simulink model "pfb_fir"  (Simulink 7.0)
settings: Solver=FixedStepDiscrete  SolverMode=SingleTasking  StartTime=0.0  StopTime=10.0  RelTol=1e-3
undefined symbols (not defined in the file): pfb_coefs
libraries: xbsIndex_r4 x385
(part 19 of 27)

== system pfb_fir/fir_2/fir_tap_3/fir_coef ==
  data_in : Inport  OutDataType=sfix(16)  OutScaling=2^0
  sum_in : Inport  Port=2  OutDataType=sfix(16)  OutScaling=2^0
  sync_in : Inport  Port=3  OutDataType=sfix(16)  OutScaling=2^0
  c_gen : Subsystem  mask(Coefficient Generator){coefs=[0.999999547662946;0.999995928971626;0.999988691616268;0.999977835651433;0.999963361158965;0.999945268247983;0.999923557054889;0.99989822774336;0.999869280504348;0.999836715556079;0.999800533144051;0.99976073354103;0.999717317047049;0.999670283989403;0.999619634722648;0.999565369628596;0.999507489116311;0.999445993622108;0.999380883609544;0.999312159569415;0.999239822019754;0.999163871505822;0.999084308600105;0.999001133902306;0.998914348039344;0.998823951665339;0.998729945461616;0.99863233013669;0.998531106426262;0.998426275093213;0.998317836927595;0.998205792746621;0.998090143394661;0.997970889743233;0.99784803269099;0.997721573163716;0.997591512114315;0.997457850522799;0.997320589396285;0.997179729768976;0.997035272702159;0.99688721928419;0.996735570630482;0.996580327883498;0.996421492212737;0.996259064814724;0.996093046912996;0.99592343975809;0.995750244627533;0.995573462825828;0.99539309568444;0.995209144561783;0.995021610843209;0.994830495940991;0.99463580129431;0.994437528369243;0.994235678658745;0.994030253682635;0.993821254987582;0.993608684147091;0.993392542761483;0.993172832457882;0.992949554890201;0.99272271173912;0.992492304712073;0.992258335543232;0.992020805993488;0.991779717850431;0.991535072928337;0.991286873068149;0.991035120137455;0.990779816030475;0.990520962668036;0.990258561997559;0.989992615993036;0.989723126655011;0.989450096010561;0.989173526113274;0.988893419043231;0.988609776906985;0.988322601837537;0.98803189599432;0.987737661563173;0.987439900756322;0.987138615812356;0.986833808996206;0.986525482599124;0.986213638938657;0.985898280358627;0.985579409229105;0.98525702794639;0.984931138932984;0.984601744637569;0.984268847534979;0.98393245012618;0.983592554938246;0.983249164524326;0.98290228146363;0.982551908361392;0.982198047848854;0.981840702583234;0.9814798752477;0.981115568551347;0.980747785229165;0.980376528042017;0.98000179977661;0.979623603245462;0.979241941286885;0.978856816764947;0.978468232569446;0.978076191615887;0.977680696845445;0.977281751224942;0.976879357746813;0.97647351942908;0.976064239315321;0.975651520474639;0.975235366001631;0.97481577901636;0.974392762664321;0.973966320116415;0.973536454568909;0.973103169243412;0.972666467386842;0.972226352271389;0.971782827194488;0.971335895478783;0.970885560472097;0.970431825547395;0.969974694102756;0.969514169561332;0.969050255371323;0.968582955005935;0.96811227196335;0.967638209766689;0.967160771963981;0.966679962128122;0.966195783856846;0.965708240772684;0.965217336522932;0.964723074779614;0.964225459239442;0.963724493623787;0.963220181678634;0.962712527174551;0.962201533906649;0.961687205694544;0.961169546382321;0.960648559838497;0.960124249955978;0.959596620652025;0.959065675868214;0.958531419570396;0.95799385574866;0.957452988417292;0.956908821614734;0.956361359403548;0.955810605870372;0.955256565125884;0.954699241304754;0.954138638565613;0.953574761091004;0.953007613087343;0.952437198784881;0.951863522437655;0.951286588323455;0.950706400743774;0.950122964023769;0.949536282512219;0.948946360581481;0.948353202627446;0.947756813069498;0.947157196350468;0.946554356936591;0.945948299317464;0.945339028005997;0.944726547538374;0.944110862474005;0.943491977395482;0.942869896908532;0.942244625641977;0.941616168247679;0.940984529400506;0.940349713798277;0.939711726161716;0.939070571234412;0.938426253782768;0.937778778595951;0.937128150485851;0.936474374287031;0.935817454856679;0.935157397074559;0.934494205842967;0.933827886086677;0.933158442752899;0.932485880811225;0.931810205253583;0.931131421094187;0.930449533369489;0.929764547138127;0.929076467480875;0.928385299500598;0.927691048322198;0.92699371909256;0.926293316980511;0.925589847176761;0.924883314893854;0.924173725366119;0.923461083849616;0.922745395622088;0.922026665982904;0.92130490025301;0.920580103774877;0.919852281912448;0.919121440051086;0.918387583597519;0.91765071797979;0.9169108486472;0.916167981070258;0.915422120740627;0.914673273171068;0.913921443895387;0.913166638468382 ...(+14460 chars)], n_bits=9, bin_pt=8, log2_cpc=0, use_bram=on}
      mask prompts: coefs "Coefficients"; n_bits "Number of Bits"; bin_pt "Binary Point"; log2_cpc "Log2 Cycles per Coefficient"; use_bram "Use BRAM"
      mask help: A coefficient generator.
      settings: AttributesFormatString=|
      | 1024 coefs in bram
      | 9_8 out/1
      mask Help:
      | <pre>
      | Description::
      | 
      | A coefficient generator.
      | 
      | Mask Parameters::
      | 
      | Coefficiants (coefs): The coefficients to output.  These should be specified as doubles.
      | They will be rounded/saturated according to the specified number of bits (n_bits)
      | and binary point (bin_pt).
      | 
      | Number of Coefficient Bits (n_bits): The number of bits used for the fixed point binary
      | representation of the coefficients.
      | 
      | Coefficient Binary Point (bin_pt): The binary point of the fixed point binary representation
      | of the coefficients.
      | 
      | Log2 Cycles per Coefficient (log2_cpc): The log2 value of the number of cycles per coefficient.
      | Must be a non-negative integer (i.e. cycles per coefficient must be a power of 2).
      | 
      | Use BRAM (use_bram): Check this checkbox to store coefficients in BRAM.
      | If unchecked, the coefficients will be sored in distributed memory (i.e. slices).
      | </pre>
  data_delay : xbsIndex_r4/Delay  en=off  latency=1  dbl_ovrd=off  reg_retiming=off  block_type=delay
      settings: xl_area=[0, 0, 0, 0, 0, 0, 0]
  sum_delay : xbsIndex_r4/Delay  en=off  latency=1  dbl_ovrd=off  reg_retiming=off  block_type=delay
      settings: xl_area=[0, 0, 0, 0, 0, 0, 0]
  sync_delay : xbsIndex_r4/Delay  en=off  latency=1  dbl_ovrd=off  reg_retiming=off  block_type=delay
      settings: xl_area=[0, 0, 0, 0, 0, 0, 0]
  data_out : Outport  OutDataType=sfix(16)  OutScaling=2^0
  sum_out : Outport  Port=2  OutDataType=sfix(16)  OutScaling=2^0
  coef : Outport  Port=3  OutDataType=sfix(16)  OutScaling=2^0
  sync_out : Outport  Port=4  OutDataType=sfix(16)  OutScaling=2^0
  wires:
  c_gen/1(coef_out) -> coef/1
  sum_delay/1 -> sum_out/1
  sum_in/1 -> sum_delay/1
  sync_in/1 -> c_gen/1(sync_in), sync_delay/1
  sync_delay/1 -> sync_out/1
  data_delay/1 -> data_out/1
  data_in/1 -> data_delay/1

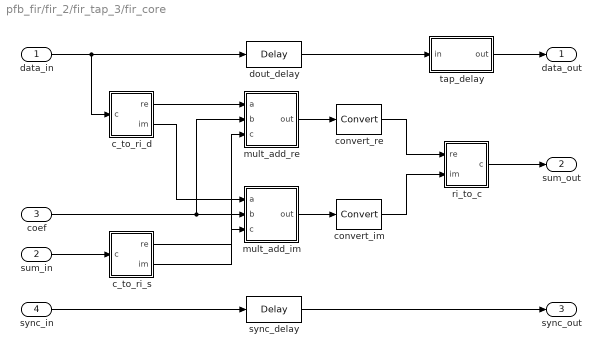
== system pfb_fir/fir_2/fir_tap_3/fir_core ==
  data_in : Inport  OutDataType=sfix(16)  OutScaling=2^0
  sum_in : Inport  Port=2  OutDataType=sfix(16)  OutScaling=2^0
  coef : Inport  Port=3  OutDataType=sfix(16)  OutScaling=2^0
  sync_in : Inport  Port=4  OutDataType=sfix(16)  OutScaling=2^0
  c_to_ri_d : Subsystem  mask(Complex to Real-Imag){n_bits=8, bin_pt=7}
      mask prompts: n_bits "Bit Width"; bin_pt "Binary Point"
      mask help: Outputs real and imaginary components of a complex input.
      settings: AttributesFormatString=8_7 r/i
      mask Help:
      | <pre>
      | Description::
      | 
      | Outputs real and imaginary components of a complex input.
      | Useful for simplifying interconnects.
      | See also: Real-Imag to Complex (ri_to_c)
      | 
      | Mask Parameters::
      | 
      | Bit Width (n_bits): Specifies the width of the real/imaginary components.
      | Assumed equal for both components.
      | 
      | Binary Point (bin_pt): Specifies the binary point location in the real/imaginary components.
      | Assumed equal for both components.
      | </pre>
  c_to_ri_s : Subsystem  mask(Complex to Real-Imag){n_bits=17, bin_pt=15}
      mask prompts: n_bits "Bit Width"; bin_pt "Binary Point"
      mask help: Outputs real and imaginary components of a complex input.
      settings: AttributesFormatString=17_15 r/i
      mask Help:
      | <pre>
      | Description::
      | 
      | Outputs real and imaginary components of a complex input.
      | Useful for simplifying interconnects.
      | See also: Real-Imag to Complex (ri_to_c)
      | 
      | Mask Parameters::
      | 
      | Bit Width (n_bits): Specifies the width of the real/imaginary components.
      | Assumed equal for both components.
      | 
      | Binary Point (bin_pt): Specifies the binary point location in the real/imaginary components.
      | Assumed equal for both components.
      | </pre>
  convert_im : xbsIndex_r4/Convert  arith_type="Signed  (2's comp)"  n_bits=17  bin_pt=15  quantization=Truncate  overflow=Wrap  latency=0  dbl_ovrd=off  pipeline=on  block_type=convert
      settings: xl_area=[0, 0, 0, 0, 0, 0, 0]  block_version=10.1.3
  convert_re : xbsIndex_r4/Convert  arith_type="Signed  (2's comp)"  n_bits=17  bin_pt=15  quantization=Truncate  overflow=Wrap  latency=0  dbl_ovrd=off  pipeline=on  block_type=convert
      settings: xl_area=[0, 0, 0, 0, 0, 0, 0]  block_version=10.1.3
  dout_delay : xbsIndex_r4/Delay  en=off  latency=4  dbl_ovrd=off  reg_retiming=off  block_type=delay
      settings: xl_area=[0, 0, 0, 0, 0, 0, 0]
  mult_add_im : Subsystem  mask(Multiply Add Block){mult_latency=3, add_latency=1, add_bypass=off}
      mask prompts: mult_latency "Multiplier Latency"; add_latency "Adder Latency"; add_bypass "Bypass Adder"
      mask help: A full precision multiply-add block. Produces a*b+c at its ab_c output. The add operation can be optionally bypassed.
      settings: AttributesFormatString=|
      | out = a*b+c
      | latency = 4
      mask Help:
      | <pre>
      | Description::
      | 
      | This full precision multiply-add block produces a*b+c at its ab_c output.
      | The add operation can be optionally bypassed.
      | 
      | Latency is one multiplier latency plus one adder latency (if not bypassing adder).
      | 
      | Mask Parameters::
      | 
      | Multiplier Latency (mult_latency): Latency to use for the underlying real multipliers.
      | 
      | Adder Latency (add_latency): Latency to use for the underlying real adders.
      | 
      | Bypass Adder (add_bypass): Check this checkbox to bypass the adder.
      | </pre>
  mult_add_re : Subsystem  mask(Multiply Add Block){mult_latency=3, add_latency=1, add_bypass=off}
      mask prompts: mult_latency "Multiplier Latency"; add_latency "Adder Latency"; add_bypass "Bypass Adder"
      mask help: A full precision multiply-add block. Produces a*b+c at its ab_c output. The add operation can be optionally bypassed.
      settings: AttributesFormatString=|
      | out = a*b+c
      | latency = 4
      mask Help:
      | <pre>
      | Description::
      | 
      | This full precision multiply-add block produces a*b+c at its ab_c output.
      | The add operation can be optionally bypassed.
      | 
      | Latency is one multiplier latency plus one adder latency (if not bypassing adder).
      | 
      | Mask Parameters::
      | 
      | Multiplier Latency (mult_latency): Latency to use for the underlying real multipliers.
      | 
      | Adder Latency (add_latency): Latency to use for the underlying real adders.
      | 
      | Bypass Adder (add_bypass): Check this checkbox to bypass the adder.
      | </pre>
  ri_to_c : Subsystem  mask(Real-Imag to Complex){}
      mask help: Concatenates real and imaginary inputs into a complex output.
      mask init:
      | ri_to_c_init(gcb);
      mask Help:
      | <pre>
      | Description::
      | 
      | Concatenates a real and imaginary input into a complex output.
      | Useful for simplifying interconnects.
      | See also: Complex to Real-Imag (c_to_ri)
      | 
      | Mask Parameters::
      | 
      | (N/A)
      | </pre>
  sync_delay : xbsIndex_r4/Delay  en=off  latency=4  dbl_ovrd=off  reg_retiming=off  block_type=delay
      settings: xl_area=[0, 0, 0, 0, 0, 0, 0]
  tap_delay : Subsystem  mask(BRAM Delay){delay_depth=1024, buffer_latency=}
      mask prompts: delay_depth "Delay Depth"; buffer_latency "Buffer Latency"
      mask help: A delay block that uses BRAM for its storage.
      settings: AttributesFormatString=bram depth = 1024
      mask Help:
      | <pre>
      | Description::
      | 
      | A delay block that uses BRAM for its storage.
      | 
      | Mask Parameters::
      | 
      | Delay Depth (delay_depth): The length of the delay.
      | 
      | Buffer Latency (buffer_latency): The latency of the underlying storage.
      | 
      | Buffer Latency defaults to 1 and cannot be changed via the block's dialog box.
      | Future versions may enable the setting of that parameter from the dialog.
      | </pre>
  data_out : Outport  OutDataType=sfix(16)  OutScaling=2^0
  sum_out : Outport  Port=2  OutDataType=sfix(16)  OutScaling=2^0
  sync_out : Outport  Port=3  OutDataType=sfix(16)  OutScaling=2^0
  wires:
  convert_im/1 -> ri_to_c/2(im)
  convert_re/1 -> ri_to_c/1(re)
  tap_delay/1(out) -> data_out/1
  mult_add_im/1(out) -> convert_im/1
  mult_add_re/1(out) -> convert_re/1
  c_to_ri_s/2(im) -> mult_add_im/3(c)
  c_to_ri_s/1(re) -> mult_add_re/3(c)
  sum_in/1 -> c_to_ri_s/1(c)
  coef/1 -> mult_add_re/2(b), mult_add_im/2(b)
  c_to_ri_d/2(im) -> mult_add_im/1(a)
  c_to_ri_d/1(re) -> mult_add_re/1(a)
  data_in/1 -> c_to_ri_d/1(c), dout_delay/1
  dout_delay/1 -> tap_delay/1(in)
  ri_to_c/1(c) -> sum_out/1
  sync_delay/1 -> sync_out/1
  sync_in/1 -> sync_delay/1

== system pfb_fir/fir_2/fir_tap_4/fir_coef ==
  data_in : Inport  OutDataType=sfix(16)  OutScaling=2^0
  sum_in : Inport  Port=2  OutDataType=sfix(16)  OutScaling=2^0
  sync_in : Inport  Port=3  OutDataType=sfix(16)  OutScaling=2^0
  c_gen : Subsystem  mask(Coefficient Generator){coefs=[0.000376226431598763;0.00113037704120664;0.00188679033646423;0.00264546512738635;0.00340640020282435;0.00416959433045314;0.00493504625675948;0.00570275470702945;0.00647271838533626;0.00724493597452914;0.00801940613622144;0.00879612751077952;0.00957509871731131;0.0103563183536561;0.0111397849963734;0.0119254972007329;0.0127134535007037;0.0135036524089452;0.0142960924167967;0.0150907719942678;0.0158876895900297;0.0166868436314057;0.0174882325243625;0.0182918546535009;0.0190977083820486;0.019905792051851;0.0207161039833637;0.0215286424756441;0.022343405806345;0.0231603922317064;0.0239795999865484;0.0248010272842649;0.0256246723168164;0.026450533254724;0.0272786082470629;0.0281088954214566;0.0289413928840709;0.0297760987196091;0.0306130109913055;0.0314521277409214;0.0322934469887399;0.0331369667335609;0.0339826849526973;0.0348305996019707;0.035680708615707;0.0365330099067331;0.0373875013663734;0.0382441808644464;0.0391030462492619;0.0399640953476175;0.0408273259647971;0.0416927358845677;0.0425603228691775;0.0434300846593541;0.0443020189743029;0.0451761235117054;0.0460523959477181;0.0469308339369715;0.0478114351125697;0.0486941970860893;0.0495791174475793;0.0504661937655611;0.0513554235870291;0.0522468044374499;0.0531403338207642;0.0540360092193872;0.0549338280942094;0.055833787884598;0.0567358860083988;0.0576401198619378;0.0585464868200229;0.0594549842359465;0.0603656094414881;0.0612783597469165;0.062193232440993;0.0631102247909746;0.0640293340426176;0.0649505574201807;0.0658738921264291;0.066799335342639;0.0677268842286013;0.0686565359226264;0.069588287541549;0.0705221361807334;0.0714580789140785;0.0723961127940227;0.0733362348515507;0.0742784420961991;0.0752227315160621;0.0761691000777984;0.0771175447266376;0.0780680623863875;0.0790206499594406;0.0799753043267821;0.0809320223479969;0.081890800861278;0.0828516366834338;0.0838145266098974;0.0847794674147343;0.0857464558506515;0.0867154886490061;0.0876865625198155;0.0886596741517658;0.0896348202122217;0.0906119973472373;0.091591202181565;0.0925724313186671;0.0935556813407251;0.094540948808652;0.0955282302621025;0.0965175222194845;0.0975088211779706;0.0985021236135104;0.0994974259808421;0.100494724713505;0.10149401622385;0.102495296903059;0.103498563121147;0.104503811226986;0.105511037548312;0.106520238391741;0.107531410042783;0.108544548765853;0.109559650804292;0.110576712380376;0.111595729695331;0.112616698929352;0.113639616241614;0.114664477770291;0.11569127963257;0.116720017924666;0.117750688721843;0.118783288078423;0.11981781202781;0.120854256582503;0.121892617734113;0.122932891453382;0.123975073690202;0.125019160373628;0.126065147411903;0.12711303069247;0.128162806081993;0.129214469426379;0.13026801655079;0.131323443259671;0.132380745336762;0.133439918545122;0.134500958627148;0.135563861304595;0.136628622278597;0.137695237229687;0.138763701817818;0.139834011682386;0.140906162442248;0.141980149695748;0.143055969020734;0.144133615974584;0.145213086094228;0.146294374896168;0.147377477876504;0.148462390510953;0.149549108254878;0.150637626543306;0.151727940790955;0.152820046392257;0.153913938721383;0.155009613132265;0.156107064958625;0.157206289513996;0.158307282091748;0.159410037965114;0.160514552387217;0.161620820591094;0.162728837789721;0.163838599176042;0.164950099922995;0.166063335183536;0.167178300090671;0.168294989757478;0.169413399277137;0.170533523722959;0.171655358148411;0.172778897587147;0.173904137053034;0.175031071540182;0.176159696022971;0.177290005456083;0.178421994774532;0.179555658893686;0.180690992709306;0.181827991097572;0.182966648915113;0.184106960999035;0.185248922166959;0.186392527217044;0.187537770928023;0.188684648059233;0.189833153350645;0.190983281522898;0.192135027277332;0.193288385296015;0.194443350241782;0.195599916758264;0.196758079469921;0.197917832982076;0.199079171880949;0.200242090733689;0.201406584088409;0.202572646474221;0.203740272401268;0.204909456360757;0.206080192825002;0.207252476247449;0.208426301062716;0.209601661686629 ...(+14467 chars)], n_bits=9, bin_pt=8, log2_cpc=0, use_bram=on}
      mask prompts: coefs "Coefficients"; n_bits "Number of Bits"; bin_pt "Binary Point"; log2_cpc "Log2 Cycles per Coefficient"; use_bram "Use BRAM"
      mask help: A coefficient generator.
      settings: AttributesFormatString=|
      | 1024 coefs in bram
      | 9_8 out/1
      mask Help:
      | <pre>
      | Description::
      | 
      | A coefficient generator.
      | 
      | Mask Parameters::
      | 
      | Coefficiants (coefs): The coefficients to output.  These should be specified as doubles.
      | They will be rounded/saturated according to the specified number of bits (n_bits)
      | and binary point (bin_pt).
      | 
      | Number of Coefficient Bits (n_bits): The number of bits used for the fixed point binary
      | representation of the coefficients.
      | 
      | Coefficient Binary Point (bin_pt): The binary point of the fixed point binary representation
      | of the coefficients.
      | 
      | Log2 Cycles per Coefficient (log2_cpc): The log2 value of the number of cycles per coefficient.
      | Must be a non-negative integer (i.e. cycles per coefficient must be a power of 2).
      | 
      | Use BRAM (use_bram): Check this checkbox to store coefficients in BRAM.
      | If unchecked, the coefficients will be sored in distributed memory (i.e. slices).
      | </pre>
  data_delay : xbsIndex_r4/Delay  en=off  latency=1  dbl_ovrd=off  reg_retiming=off  block_type=delay
      settings: xl_area=[0, 0, 0, 0, 0, 0, 0]
  sum_delay : xbsIndex_r4/Delay  en=off  latency=1  dbl_ovrd=off  reg_retiming=off  block_type=delay
      settings: xl_area=[0, 0, 0, 0, 0, 0, 0]
  sync_delay : xbsIndex_r4/Delay  en=off  latency=1  dbl_ovrd=off  reg_retiming=off  block_type=delay
      settings: xl_area=[0, 0, 0, 0, 0, 0, 0]
  data_out : Outport  OutDataType=sfix(16)  OutScaling=2^0
  sum_out : Outport  Port=2  OutDataType=sfix(16)  OutScaling=2^0
  coef : Outport  Port=3  OutDataType=sfix(16)  OutScaling=2^0
  sync_out : Outport  Port=4  OutDataType=sfix(16)  OutScaling=2^0
  wires:
  c_gen/1(coef_out) -> coef/1
  sum_delay/1 -> sum_out/1
  sum_in/1 -> sum_delay/1
  sync_in/1 -> c_gen/1(sync_in), sync_delay/1
  sync_delay/1 -> sync_out/1
  data_delay/1 -> data_out/1
  data_in/1 -> data_delay/1
